simulink model "B_MotorSpeed_Task3"  (R2021b)
settings: Solver=VariableStepAuto  StartTime=0.0  StopTime=20  FixedStep=Ts  RelTol=1e-3
PreLoadFcn:
  | clear
  | load('MotorSpeedTask3_Parameters.mat')
  | load('PID_CalibrationValues_Motor.mat')
PostLoadFcn:
  | load('MotorSpeedTask3_Parameters.mat')
  | load('PID_CalibrationValues_Motor.mat')
undefined symbols (not defined in the file): b, J, Ke, Kt, L, R
CloseFcn:
  | clear;
settings Model: Creator=vigne  LastModifiedBy=vigne
settings OptimizationCC: UseDivisionForNetSlopeComputation=on

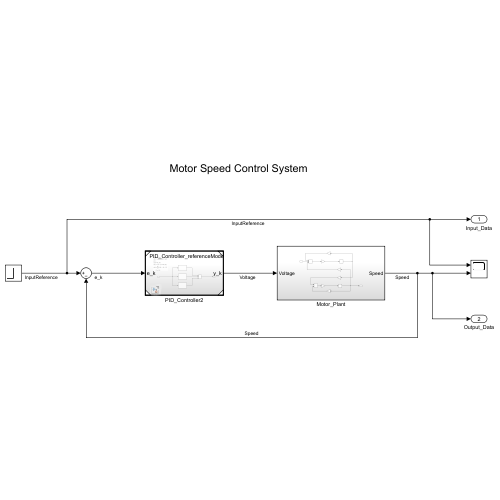
[thumbnail: Simulink's stored preview of the top-level diagram]
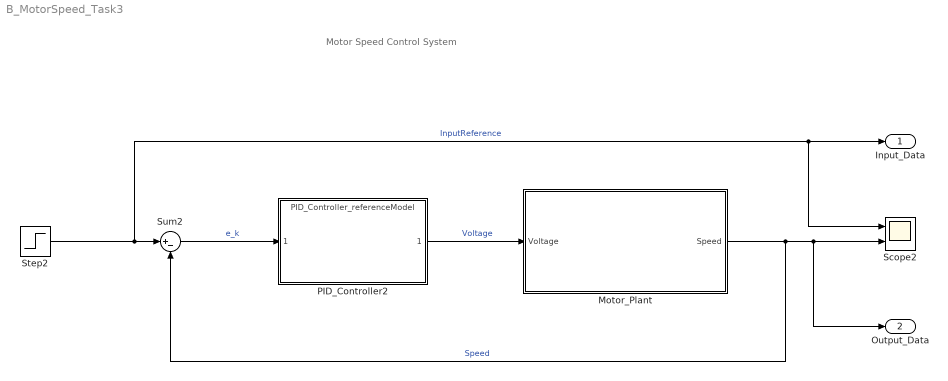
== system B_MotorSpeed_Task3 ==
  note: Motor Speed Control System
  Motor_Plant : Subsystem
  PID_Controller2 : ModelReference  ModelNameDialog=PID_Controller_referenceModel.slx  ModelReferenceVersion=1.13
  Scope2 : Scope  NumInputPorts=2
  Step2 : Step  After=100  SampleTime=0
  Sum2 : Sum  Inputs=|+-
  Input_Data : Outport
  Output_Data : Outport  Port=2
  wires:
  Sum2/1 -> PID_Controller2/1  "e_k"
  Motor_Plant/1(Speed) -> Sum2/2, Output_Data/1, Scope2/2  "Speed"
  Step2/1 -> Scope2/1, Input_Data/1, Sum2/1  "InputReference"
  PID_Controller2/1 -> Motor_Plant/1(Voltage)  "Voltage"

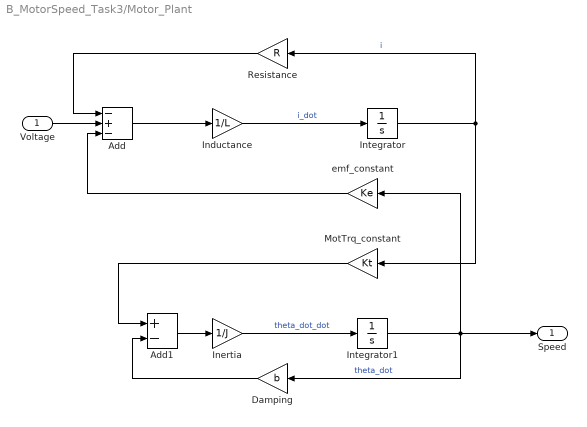
== system B_MotorSpeed_Task3/Motor_Plant ==
  Voltage : Inport
  Add : Sum  Inputs=-+-
  Add1 : Sum  Inputs=+-
  Damping : Gain  Gain=b
  Inductance : Gain  Gain=1/L
  Inertia : Gain  Gain=1/J
  Integrator : Integrator
  Integrator1 : Integrator
  MotTrq_constant : Gain  Gain=Kt
  Resistance : Gain  Gain=R
  emf_constant : Gain  Gain=Ke
  Speed : Outport
  wires:
  Integrator/1 -> Resistance/1, MotTrq_constant/1  "i"
  Add1/1 -> Inertia/1
  Add/1 -> Inductance/1
  Voltage/1 -> Add/2
  Resistance/1 -> Add/1
  MotTrq_constant/1 -> Add1/1
  Inductance/1 -> Integrator/1  "i_dot"
  Integrator1/1 -> Speed/1, emf_constant/1, Damping/1  "theta_dot"
  Inertia/1 -> Integrator1/1  "theta_dot_dot"
  emf_constant/1 -> Add/3
  Damping/1 -> Add1/2
